simulink model "train_system"  (R2022a)
settings: Solver=VariableStepAuto  StartTime=0.0  StopTime=10.0  RelTol=1e-3
settings Model: Creator=kasturkoul  LastModifiedBy=kasturkoul

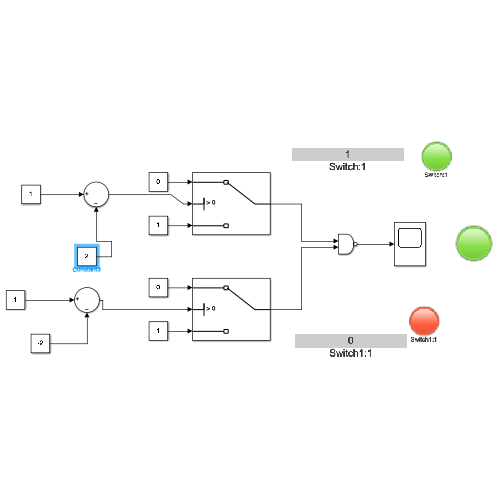
[thumbnail: Simulink's stored preview of the top-level diagram]
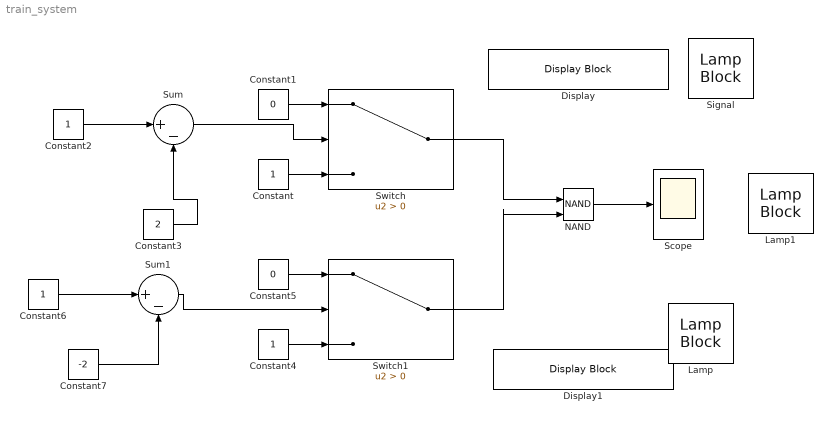
== system train_system ==
  Constant{,2,4,6} (4 alike) : Constant
  Constant1 : Constant  Value=0
  Constant3 : Constant  Value=2
  Constant5 : Constant  Value=0
  Constant7 : Constant  Value=-2
  Display : DisplayBlock  LabelPosition=Bottom  Transparency=1
  Display1 : DisplayBlock  LabelPosition=Bottom  Transparency=1
  Lamp : LampBlock  LabelPosition=Bottom
  Lamp1 : LampBlock  LabelPosition=Hide
  NAND : Logic  Operator=NAND  IconShape=distinctive  AllPortsSameDT=off  OutDataTypeStr=boolean
  Scope : Scope
  Signal : LampBlock  LabelPosition=Bottom
  Sum : Sum  Inputs=|+-
  Sum1 : Sum  Inputs=|+-
  Switch : Switch  Criteria=u2 > Threshold  SaturateOnIntegerOverflow=off  InputSameDT=off
  Switch1 : Switch  Criteria=u2 > Threshold  SaturateOnIntegerOverflow=off  InputSameDT=off
  wires:
  Switch/1 -> NAND/1
  Constant/1 -> Switch/3
  Constant1/1 -> Switch/1
  Constant2/1 -> Sum/1
  Constant3/1 -> Sum/2
  Sum/1 -> Switch/2
  Constant7/1 -> Sum1/2
  Sum1/1 -> Switch1/2
  Switch1/1 -> NAND/2
  Constant6/1 -> Sum1/1
  Constant5/1 -> Switch1/1
  Constant4/1 -> Switch1/3
  NAND/1 -> Scope/1
